simulink model "threephaseinverter_SRF"  (R2023b)
settings: Solver=VariableStepAuto  StartTime=0.0  StopTime=30  RelTol=1e-3
libraries: spsGroundLib x13, spsSeriesRLCBranchLib x12, spsBreakerLib x9, spsIGBTDiodeLib x6, spsSeriesRLCLoadLib x6, spsCurrentMeasurementLib x5, spsVoltageMeasurementLib x4, eeGeneralControl x4, dspsigops x3, slpidlib x2, spsAlphaBetaZerotodq0Lib x2, spsabctoAlphaBetaZeroLib x2
settings Model: Creator=Jia Yee Wong  LastModifiedBy=Jia Yee Wong
settings SFSimCC: SimCustomHeaderCode="#include \"referencegen.h\""  SimUserSources=referencegen.cpp;  SimUserIncludeDirs=C:\JJ\FinalYearProject  DefaultCustomCodeDeterministicFunctions=ByFunction  SimTargetLang=C++

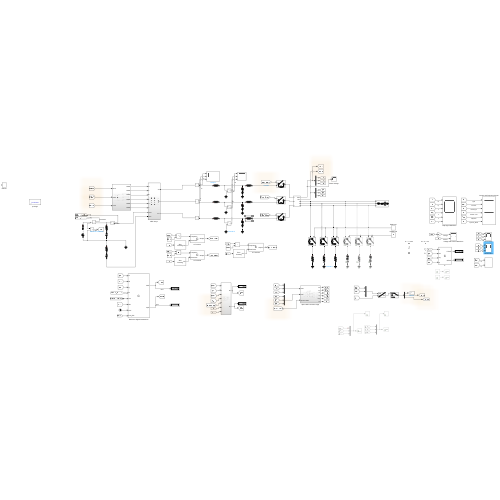
[thumbnail: Simulink's stored preview of the top-level diagram]
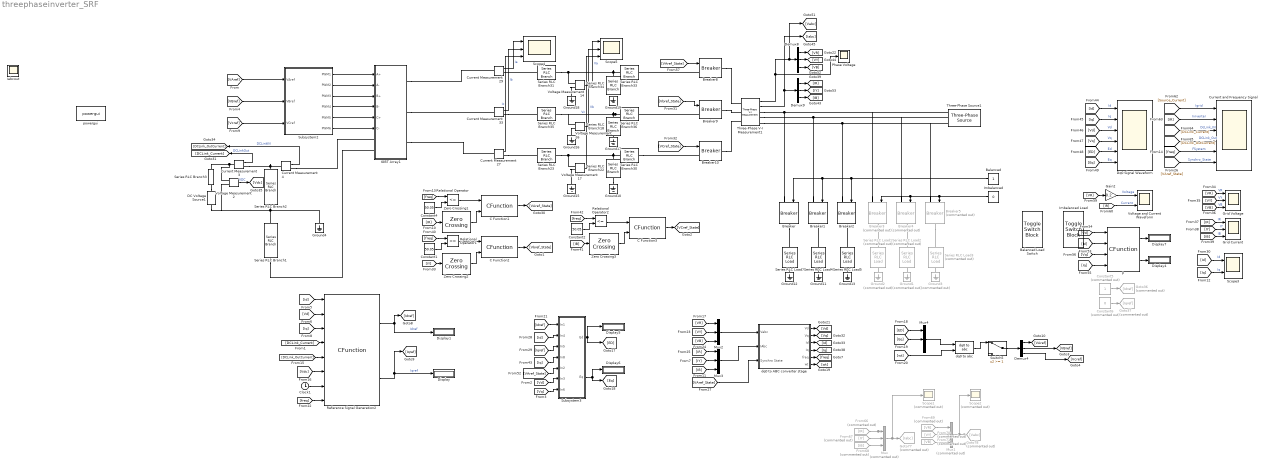
== system threephaseinverter_SRF ==
  Balanced : Constant
  Balanced Load Switch : ToggleSwitchBlock
      settings: Values={{'Off', 'On'}, [0 1]}
  Breaker : spsBreakerLib/Breaker  InitialState=0  SwitchingTimes="[1/60  5/60]"  External=on  BreakerResistance=0.01  SnubberResistance=1e6  SnubberCapacitance=inf  Measurements=None  MoreParameters=on  NoBreakLoop=off
  Breaker1 : spsBreakerLib/Breaker  InitialState=0  SwitchingTimes="[1/60  5/60]"  External=on  BreakerResistance=0.01  SnubberResistance=1e6  SnubberCapacitance=inf  Measurements=None  MoreParameters=on  NoBreakLoop=off
  Breaker10 : spsBreakerLib/Breaker  InitialState=0  SwitchingTimes="[1/60  5/60]"  External=on  BreakerResistance=0.00001  SnubberResistance=30  SnubberCapacitance=47e-9  Measurements=None  MoreParameters=on  NoBreakLoop=off
  Breaker2 : spsBreakerLib/Breaker  InitialState=0  SwitchingTimes="[1/60  5/60]"  External=on  BreakerResistance=0.01  SnubberResistance=1e6  SnubberCapacitance=inf  Measurements=None  MoreParameters=on  NoBreakLoop=off
  Breaker3 : spsBreakerLib/Breaker  Commented=on  InitialState=0  SwitchingTimes="[1/60  5/60]"  External=on  BreakerResistance=0.01  SnubberResistance=1e6  SnubberCapacitance=inf  Measurements=None  MoreParameters=on  NoBreakLoop=off
  Breaker4 : spsBreakerLib/Breaker  Commented=on  InitialState=0  SwitchingTimes="[1/60  5/60]"  External=on  BreakerResistance=0.01  SnubberResistance=1e6  SnubberCapacitance=inf  Measurements=None  MoreParameters=on  NoBreakLoop=off
  Breaker5 : spsBreakerLib/Breaker  Commented=on  InitialState=0  SwitchingTimes="[1/60  5/60]"  External=on  BreakerResistance=0.01  SnubberResistance=1e6  SnubberCapacitance=inf  Measurements=None  MoreParameters=on  NoBreakLoop=off
  Breaker8 : spsBreakerLib/Breaker  InitialState=0  SwitchingTimes="[1/60  5/60]"  External=on  BreakerResistance=0.00001  SnubberResistance=30  SnubberCapacitance=47e-9  Measurements=None  MoreParameters=on  NoBreakLoop=off
  Breaker9 : spsBreakerLib/Breaker  InitialState=0  SwitchingTimes="[1/60  5/60]"  External=on  BreakerResistance=0.00001  SnubberResistance=30  SnubberCapacitance=47e-9  Measurements=None  MoreParameters=on  NoBreakLoop=off
  C Function1 : CFunction  OutputCode=|  SampleTime=1/50000
      | if(Frequency == true && ZeroCross == 1){
      |     Output = 1;}
      | else if(Frequency == false){
      |         Output = 0;}
  C Function2 : CFunction  OutputCode=|  SampleTime=1/50000
      | if(Frequency == true && ZeroCross == 1){
      |     Output = 1;}
      | else if(Frequency == false){
      |         Output = 0;}
  C Function3 : CFunction  OutputCode=|  SampleTime=1/50000
      | if(Frequency == true && ZeroCross == 1){
      |     Output = 1;}
      | else if(Frequency == false){
      |         Output = 0;}
  Clock1 : Clock
  Constant1 : Constant  Value=50.05  SampleTime=1/50000
  Constant2 : Constant  Value=50.05  SampleTime=1/50000
  Constant4 : Constant  Value=50.05  SampleTime=1/50000
  Constant5 : Constant  Commented=on
  Constant6 : Constant  Commented=on  Value=0
  Current Measurement{3..4,27,29,33} (5 alike) : spsCurrentMeasurementLib/Current Measurement  PhasorSimulation=off  OutputType=Complex  PSBequivalent=0
  Current and Frequency Signal : Scope  NumInputPorts=6
  DC Voltage Source1 : spsDCVoltageSourceLib/DC Voltage Source  Amplitude=400  Measurements=None
  Demux4 : Demux  Outputs=3
  Demux8 : Demux  Outputs=3
  Demux9 : Demux  Outputs=3
  Display{,1,4..7} (6 alike) : Display
  Dq0 Signal Waveform : Scope  NumInputPorts=6
  From66 : From  Commented=on  GotoTag=IR
  From67 : From  Commented=on  GotoTag=IY
  From68 : From  Commented=on  GotoTag=IB
  From69 : From  Commented=on  GotoTag=VR
  From70 : From  Commented=on  GotoTag=VY
  From71 : From  Commented=on  GotoTag=VB
  Gain2 : Gain  Gain=0.2
  Goto36 : Goto  Commented=on  GotoTag=Idref
  Goto37 : Goto  Commented=on  GotoTag=Iqref
  Goto77 : Goto  Commented=on  GotoTag=Iabc
  Goto78 : Goto  Commented=on  GotoTag=Vabc
  Grid Current : Scope  NumInputPorts=3
  Grid Voltage : Scope  NumInputPorts=3
  Ground1 : spsGroundLib/Ground  Commented=on  LConnTagsString=a
  Ground{4,10..13,15..19} (10 alike) : spsGroundLib/Ground  LConnTagsString=a
  Ground2 : spsGroundLib/Ground  Commented=on  LConnTagsString=a
  Ground3 : spsGroundLib/Ground  Commented=on  LConnTagsString=a
  IGBT Array1 : Subsystem
  Iabcout : Scope
  Imbalanced : Constant  Value=0
  Imbalanced Load : ToggleSwitchBlock
      settings: Values={{'Off', 'On'}, [0 1]}
  Mux : Mux  Commented=on  Inputs=3
  Mux1 : Mux  Commented=on  Inputs=3
  Mux2 : Mux  Inputs=3
  Mux3 : Mux  Inputs=3
  Mux4 : Mux  Inputs=3
  P : CFunction  OutputCode=|
      | PTotal = Id*Vd;
      | QTotal = Id*Vq-Vq*Id;
  Phase Voltage : Scope
  Reference Signal Generation2 : CFunction  OutputCode=|  StartCode=|  SampleTime=1/50000
      OutputCode=|
      | if(Id!=PreviousId || Iq!=PreviousIq){
      |     if(ReferenceGenTrigger(Freq_PLL)){
      |         Idref=IdrefCalc(CLK,Vd,Iin,Iout, Vdc, Vdc);
      |   //Idref =1;
      |    Iqref=0;
      |    PreviousId=Id;
      |    PreviousIq=Iq;
      |    }
      |   
      | } else { Idref = 0; Iqref = 0;}
      StartCode=|
      | PreviousIq =0;
      | PreviousId =0;
  Relational Operator : RelationalOperator  Operator=<=  OutDataTypeStr=boolean  RndMeth=Simplest  InputSameDT=off
  Relational Operator1 : RelationalOperator  Operator=<=  OutDataTypeStr=boolean  RndMeth=Simplest  InputSameDT=off
  Relational Operator2 : RelationalOperator  Operator=<=  OutDataTypeStr=boolean  RndMeth=Simplest  InputSameDT=off
  Scope1 : Scope  Commented=on
  Scope2 : Scope  Commented=on
  Scope3 : Scope  NumInputPorts=2
  Scope4 : Scope  NumInputPorts=3
  Scope5 : Scope  NumInputPorts=3
  Series RLC Branch1 : spsSeriesRLCBranchLib/Series RLC Branch  LConnTagsString=__new0  RConnTagsString=__new0  BranchType=RC  Resistance=1  Inductance=0  SetiL0=off  InitialCurrent=0  Capacitance=47e-3  Setx0=off  InitialVoltage=300  Measurements=None
  Series RLC Branch18 : spsSeriesRLCBranchLib/Series RLC Branch  LConnTagsString=__new0  RConnTagsString=__new0  BranchType=RC  Resistance=120  Inductance=100e-6  SetiL0=off  InitialCurrent=0  Capacitance=5.526e-6  Setx0=off  InitialVoltage=0  Measurements=None
  Series RLC Branch2 : spsSeriesRLCBranchLib/Series RLC Branch  LConnTagsString=__new0  RConnTagsString=__new0  BranchType=RC  Resistance=1  Inductance=0  SetiL0=off  InitialCurrent=0  Capacitance=47e-3  Setx0=off  InitialVoltage=300  Measurements=None
  Series RLC Branch22 : spsSeriesRLCBranchLib/Series RLC Branch  LConnTagsString=__new0  RConnTagsString=__new0  BranchType=RC  Resistance=120  Inductance=100e-6  SetiL0=off  InitialCurrent=0  Capacitance=5.526e-6  Setx0=off  InitialVoltage=0  Measurements=None
  Series RLC Branch23 : spsSeriesRLCBranchLib/Series RLC Branch  LConnTagsString=__new0  RConnTagsString=__new0  BranchType=L  Resistance=1  Inductance=20.4e-3  SetiL0=off  InitialCurrent=0  Capacitance=1e-6  Setx0=off  InitialVoltage=0  Measurements=None
  Series RLC Branch3 : spsSeriesRLCBranchLib/Series RLC Branch  LConnTagsString=__new0  RConnTagsString=__new0  BranchType=RL  Resistance=100  Inductance=0  SetiL0=off  InitialCurrent=0  Capacitance=1e-6  Setx0=off  InitialVoltage=0  Measurements=None
  Series RLC Branch30 : spsSeriesRLCBranchLib/Series RLC Branch  LConnTagsString=__new0  RConnTagsString=__new0  BranchType=L  Resistance=1  Inductance=148.336e-6  SetiL0=off  InitialCurrent=0  Capacitance=1e-6  Setx0=off  InitialVoltage=0  Measurements=None
  Series RLC Branch31 : spsSeriesRLCBranchLib/Series RLC Branch  LConnTagsString=__new0  RConnTagsString=__new0  BranchType=L  Resistance=1  Inductance=20.4e-3  SetiL0=off  InitialCurrent=0  Capacitance=1e-6  Setx0=off  InitialVoltage=0  Measurements=None
  Series RLC Branch33 : spsSeriesRLCBranchLib/Series RLC Branch  LConnTagsString=__new0  RConnTagsString=__new0  BranchType=L  Resistance=1  Inductance=148.336e-6  SetiL0=off  InitialCurrent=0  Capacitance=1e-6  Setx0=off  InitialVoltage=0  Measurements=None
  Series RLC Branch34 : spsSeriesRLCBranchLib/Series RLC Branch  LConnTagsString=__new0  RConnTagsString=__new0  BranchType=RC  Resistance=120  Inductance=100e-6  SetiL0=off  InitialCurrent=0  Capacitance=5.526e-6  Setx0=off  InitialVoltage=0  Measurements=None
  Series RLC Branch35 : spsSeriesRLCBranchLib/Series RLC Branch  LConnTagsString=__new0  RConnTagsString=__new0  BranchType=L  Resistance=1  Inductance=20.4e-3  SetiL0=off  InitialCurrent=0  Capacitance=1e-6  Setx0=off  InitialVoltage=0  Measurements=None
  Series RLC Branch36 : spsSeriesRLCBranchLib/Series RLC Branch  LConnTagsString=__new0  RConnTagsString=__new0  BranchType=L  Resistance=1  Inductance=148.336e-6  SetiL0=off  InitialCurrent=0  Capacitance=1e-6  Setx0=off  InitialVoltage=0  Measurements=None
  Series RLC Load1 : spsSeriesRLCLoadLib/Series RLC Load  Commented=on  LConnTagsString=a  RConnTagsString=__new0  NominalVoltage=240  NominalFrequency=50  ActivePower=10e3  InductivePower=300  CapacitivePower=200  Setx0=off  InitialVoltage=240  SetiL0=off  InitialCurrent=10  Measurements=None  LoadType=constant PQ
  Series RLC Load2 : spsSeriesRLCLoadLib/Series RLC Load  Commented=on  LConnTagsString=a  RConnTagsString=__new0  NominalVoltage=240  NominalFrequency=50  ActivePower=10e3  InductivePower=0  CapacitivePower=0  Setx0=off  InitialVoltage=240  SetiL0=off  InitialCurrent=10  Measurements=None  LoadType=constant PQ
  Series RLC Load3 : spsSeriesRLCLoadLib/Series RLC Load  Commented=on  LConnTagsString=a  RConnTagsString=__new0  NominalVoltage=240  NominalFrequency=50  ActivePower=5e3  InductivePower=400  CapacitivePower=0  Setx0=off  InitialVoltage=240  SetiL0=off  InitialCurrent=10  Measurements=None  LoadType=constant PQ
  Series RLC Load4 : spsSeriesRLCLoadLib/Series RLC Load  LConnTagsString=a  RConnTagsString=__new0  NominalVoltage=240  NominalFrequency=50  ActivePower=10e2  InductivePower=0  CapacitivePower=0  Setx0=off  InitialVoltage=240  SetiL0=off  InitialCurrent=10  Measurements=None  LoadType=constant PQ
  Series RLC Load5 : spsSeriesRLCLoadLib/Series RLC Load  LConnTagsString=a  RConnTagsString=__new0  NominalVoltage=240  NominalFrequency=50  ActivePower=10e2  InductivePower=0  CapacitivePower=0  Setx0=off  InitialVoltage=240  SetiL0=off  InitialCurrent=10  Measurements=None  LoadType=constant PQ
  Series RLC Load7 : spsSeriesRLCLoadLib/Series RLC Load  LConnTagsString=a  RConnTagsString=__new0  NominalVoltage=240  NominalFrequency=50  ActivePower=10e2  InductivePower=0  CapacitivePower=0  Setx0=off  InitialVoltage=240  SetiL0=off  InitialCurrent=10  Measurements=None  LoadType=constant PQ
  Subsystem2 : Subsystem
  Subsystem3 : Subsystem
  Switch5 : Switch  Threshold=1  SaturateOnIntegerOverflow=off  InputSameDT=off
  Three-Phase V-I Measurement1 : spsThreePhaseVIMeasurementLib/Three-Phase V-I Measurement  VoltageMeasurement=phase-to-phase  SetLabelV=off  LabelV=Vabc  Vpu=off  VpuLL=off  CurrentMeasurement=yes  SetLabelI=off  LabelI=Iabc  Ipu=off  Pbase=100e6  Vbase=500e3  OutputType=Complex  PhasorSimulation=off  PSBequivalent=0
  Three-Phase Source1 : spsThreePhaseSourceLib/Three-Phase Source  InternalConnection=Yg  VoltagePhases=off  Voltage=240  PhaseAngle=0  Voltage_phases=[25e3 25e3 25e3]/sqrt(3)  PhaseAngles_phases=[0 -120 +120]  Frequency=50  NonIdealSource=on  SpecifyImpedance=off  Resistance=0.001E-3  Inductance=0.001E-3  ShortCircuitLevel=100e6  BaseVoltage=240  XRratio=7  BusType=PQ  Pref=1000  Qref=0  Prefabc=[10e3, 10e3, 10e3]  Qrefabc=[0, 0, 0]  Qmin=-inf  Qmax=inf
  Voltage Measurement{2,14,16..17} (4 alike) : spsVoltageMeasurementLib/Voltage Measurement  PhasorSimulation=off  OutputType=Complex  PSBequivalent=0
  Voltage and Current Waveform : Scope  NumInputPorts=2
  Zero Crossing1 : dspsigops/Zero Crossing
  Zero Crossing2 : dspsigops/Zero Crossing
  Zero Crossing3 : dspsigops/Zero Crossing
  dq0 to ABC converter stage : Subsystem
  dq0 to abc : spsdq0toabcLib/dq0 to abc  Alignment=90 degrees behind phase A axis
  powergui : spspowerguiLib/powergui  Priority=1  SimulationMode=Continuous  SampleTime=50e-6  frequency=60  Iterations=50  frequencyindice=0  Pbase=100e6  ErrMax=1e-4  UnitsV=kV  UnitsW=MW  buscounter=0  FunctionMessages=off  echomessages=off  EnableUseOfTLC=off  CurrentSourceSwitches=off  DisableSnubberDevices=off  DisableRonSwitches=off  DisableVfSwitches=off  DisplayEquations=off  AutomaticDiscreteSolvers=off  SolverType=Tustin/Backward Euler (TBE)  Interpol=off  ExternalGateDelay=off  methode=off  Ts=100  x0status=blocks  SPID=on  SwTol=0  HookPort=off  NonlinearTolerance=1e-4  nMaxIteration=100  ContinueOnMaxIteration=off  RestoreLinks=warning  ResistiveCurrentMeasurement=off  Frange=[0:2:500]  Ylog=off  Xlog=on  ShowGrid=off  save=off  variable=ZData  structure=0  ZoomFFT=off  StartTime=0.0  cycles=1  DisplayStyle=1  fundamental=60  FreqAxis=off  MaxFrequency=1000  frequencyindicesteady=1  RmsSteady=1  display=off
  wires:
  Mux/1 -> Scope1/1, Goto77/1
  From68/1 -> Mux/3
  From67/1 -> Mux/2
  From66/1 -> Mux/1
  From70/1 -> Mux1/2
  From69/1 -> Mux1/1
  From71/1 -> Mux1/3
  Mux1/1 -> Scope2/1, Goto78/1
  Demux9/3 -> [IB]
  Demux9/1 -> [IR]
  Demux8/2 -> [VY]
  Demux8/1 -> [VR]
  Three-Phase V-I Measurement1/2 -> [Iabc], Demux9/1
  [VAref_State] -> Breaker8/1
  [Vbref_State] -> Breaker9/1
  Three-Phase V-I Measurement1/1 -> Phase Voltage/1, [Vabc], Demux8/1
  Demux8/3 -> [VB]
  Voltage Measurement16/1 -> Scope5/2  "Vb"
  Voltage Measurement14/1 -> Scope5/1  "Va"
  [VCref_State] -> Breaker10/1
  Demux9/2 -> [IY]
  Balanced/1 -> Breaker2/1, Breaker1/1, Breaker/1
  Voltage Measurement17/1 -> Scope5/3  "Vc"
  Imbalanced/1 -> Breaker5/1, Breaker4/1, Breaker3/1
  Current Measurement27/1 -> Scope4/3  "Ic"
  Current Measurement33/1 -> Scope4/2  "Ib"
  Current Measurement29/1 -> Scope4/1  "Ia"
  Subsystem2/1(PWM1) -> IGBT Array1/1(A+)
  Subsystem2/2(PWM2) -> IGBT Array1/2(A-)
  Subsystem2/3(PWM3) -> IGBT Array1/3(B+)
  Subsystem2/4(PWM4) -> IGBT Array1/4(B-)
  Subsystem2/5(PWM5) -> IGBT Array1/5(C+)
  Subsystem2/6(PWM6) -> IGBT Array1/6(C-)
  Current Measurement4/1 -> [DCLink_OutCurrent]  "DCLinkIN"
  Current Measurement3/1 -> [DCLink_Current]  "DCLinkOut"
  Voltage Measurement2/1 -> [Vdc]  "VDC"
  Reference Signal Generation2/1 -> Display1/1, [Idref]  "Idref"
  [Id] -> Reference Signal Generation2/1
  Clock1/1 -> Reference Signal Generation2/7
  [freq] -> Reference Signal Generation2/8
  [Iq] -> Reference Signal Generation2/3
  [DCLink_OutCurrent] -> Reference Signal Generation2/5
  [Vdc] -> Reference Signal Generation2/6
  [Vd] -> Reference Signal Generation2/2
  [DCLink_Current] -> Reference Signal Generation2/4
  Reference Signal Generation2/2 -> [Iqref], Display/1  "Iqref"
  [Id] -> Subsystem3/2(In4)
  [VAref_State] -> Subsystem3/5(In2)
  [Iq] -> Subsystem3/4(In8)
  Subsystem3/2(Eq) -> [Eq], Display6/1
  Subsystem3/1(Ed) -> [ED], Display5/1
  [Vq] -> Subsystem3/7(In6)
  [Vd] -> Subsystem3/6(In3)
  [Iqref] -> Subsystem3/3(In5)
  [Idref] -> Subsystem3/1(In1)
  Mux3/1 -> dq0 to ABC converter stage/2(IAbc)
  [VB] -> Mux2/3
  dq0 to ABC converter stage/4(Iq) -> [Iq]
  [IB] -> Mux3/3
  dq0 to ABC converter stage/3(Id) -> [Id]
  dq0 to ABC converter stage/5(freq) -> [freq]
  [IR] -> Mux3/1
  dq0 to ABC converter stage/2(Vq) -> [Vq]
  Mux2/1 -> dq0 to ABC converter stage/1(Vabc)
  dq0 to ABC converter stage/1(Vd) -> [Vd]
  [VR] -> Mux2/1
  [IY] -> Mux3/2
  [VAref_State] -> dq0 to ABC converter stage/3(Synchro State)
  dq0 to ABC converter stage/6(wt) -> [wt]
  [VY] -> Mux2/2
  Switch5/1 -> Demux4/1
  [ED] -> Mux4/1
  Mux4/1 -> dq0 to abc/1
  dq0 to abc/1 -> Switch5/1
  [Eq] -> Mux4/2
  [wt] -> dq0 to abc/2
  Demux4/1 -> [VAref]
  Demux4/2 -> [VBref]
  Demux4/3 -> [Vcref]
  [Vcref] -> Subsystem2/3(VCref)
  [VBref] -> Subsystem2/2(VBref)
  [VAref] -> Subsystem2/1(VAref)
  Zero Crossing1/1 -> C Function1/2
  Constant4/1 -> Relational Operator/2
  [IR] -> Zero Crossing1/1
  Relational Operator/1 -> C Function1/1
  [freq] -> Relational Operator/1
  C Function1/1 -> [VAref_State]
  P/2 -> Display4/1
  [freq] -> Current and Frequency Signal/5  "FSystem"
  Constant5/1 -> Goto36/1
  [IR] -> Grid Current/1  "IR"
  P/1 -> Display7/1
  Constant6/1 -> Goto37/1
  [IB] -> Grid Current/3  "IB"
  [ED] -> Dq0 Signal Waveform/5  "Ed"
  [VAref_State] -> Current and Frequency Signal/6  "Synchro_State"
  [Id] -> P/2
  [DCLink_Current] -> Current and Frequency Signal/3  "DcLink_IN"
  [Vq] -> Dq0 Signal Waveform/4  "Vq"
  [VR] -> Grid Voltage/1  "VR"
  [Vd] -> Dq0 Signal Waveform/3  "Vd"
  [VR] -> Gain2/1
  [VY] -> Grid Voltage/2  "VY"
  [Vd] -> P/1
  [IR] -> Voltage and Current Waveform/2  "Current"
  [IY] -> Grid Current/2  "IY"
  [Vq] -> P/3
  [Eq] -> Dq0 Signal Waveform/6  "Eq"
  [IR] -> Current and Frequency Signal/2  "Iinverter"
  Gain2/1 -> Voltage and Current Waveform/1  "Voltage"
  [Source_Current] -> Current and Frequency Signal/1  "Igrid"
  [Iq] -> Dq0 Signal Waveform/2  "Iq"
  [VB] -> Grid Voltage/3  "VB"
  [Iq] -> Scope3/2  "Iq"
  [Id] -> Scope3/1  "Id"
  [Id] -> Dq0 Signal Waveform/1  "Id"
  [DCLink_OutCurrent] -> Current and Frequency Signal/4  "DCLink_Out"
  [Iq] -> P/4
  C Function2/1 -> [Vbref_State]
  Zero Crossing2/1 -> C Function2/2
  Constant1/1 -> Relational Operator1/2
  Relational Operator1/1 -> C Function2/1
  [IY] -> Zero Crossing2/1
  [freq] -> Relational Operator1/1
  [freq] -> Relational Operator2/1
  Zero Crossing3/1 -> C Function3/2
  Relational Operator2/1 -> C Function3/1
  [IB] -> Zero Crossing3/1
  Constant2/1 -> Relational Operator2/2
  C Function3/1 -> [VCref_State]
  connections:
  Three-Phase V-I Measurement1/RConn3 -- Three-Phase Source1/RConn3 -- Breaker5/LConn1 -- Breaker2/LConn1
  Three-Phase V-I Measurement1/RConn1 -- Three-Phase Source1/RConn1 -- Breaker3/LConn1 -- Breaker/LConn1
  Voltage Measurement17/LConn1 -- Series RLC Branch23/RConn1 -- Series RLC Branch30/LConn1 -- Series RLC Branch22/LConn1
  Voltage Measurement14/LConn1 -- Series RLC Branch31/RConn1 -- Series RLC Branch33/LConn1 -- Series RLC Branch34/LConn1
  Three-Phase V-I Measurement1/RConn2 -- Three-Phase Source1/RConn2 -- Breaker4/LConn1 -- Breaker1/LConn1
  Series RLC Branch36/LConn1 -- Voltage Measurement16/LConn1 -- Series RLC Branch35/RConn1 -- Series RLC Branch18/LConn1
  Breaker9/LConn1 -- Series RLC Branch36/RConn1
  Voltage Measurement17/LConn2 -- Ground15/LConn1
  Breaker8/LConn1 -- Series RLC Branch33/RConn1
  Ground12/LConn1 -- Series RLC Load7/RConn1
  Ground16/LConn1 -- Voltage Measurement16/LConn2
  Breaker8/RConn1 -- Three-Phase V-I Measurement1/LConn1
  Voltage Measurement14/LConn2 -- Ground18/LConn1
  Breaker9/RConn1 -- Three-Phase V-I Measurement1/LConn2
  Series RLC Load4/RConn1 -- Ground11/LConn1
  Series RLC Branch30/RConn1 -- Breaker10/LConn1
  Series RLC Branch22/RConn1 -- Ground10/LConn1
  Series RLC Load5/RConn1 -- Ground13/LConn1
  Breaker10/RConn1 -- Three-Phase V-I Measurement1/LConn3
  Current Measurement29/RConn1 -- Series RLC Branch31/LConn1
  Series RLC Branch18/RConn1 -- Ground17/LConn1
  IGBT Array1/RConn2 -- Current Measurement33/LConn1
  Current Measurement27/RConn1 -- Series RLC Branch23/LConn1
  Current Measurement33/RConn1 -- Series RLC Branch35/LConn1
  IGBT Array1/RConn3 -- Current Measurement27/LConn1
  Breaker/RConn1 -- Series RLC Load7/LConn1
  Series RLC Load4/LConn1 -- Breaker1/RConn1
  Series RLC Load5/LConn1 -- Breaker2/RConn1
  Ground2/LConn1 -- Series RLC Load1/RConn1
  Ground1/LConn1 -- Series RLC Load2/RConn1
  Breaker3/RConn1 -- Series RLC Load1/LConn1
  Ground3/LConn1 -- Series RLC Load3/RConn1
  Breaker4/RConn1 -- Series RLC Load2/LConn1
  Breaker5/RConn1 -- Series RLC Load3/LConn1
  IGBT Array1/RConn1 -- Current Measurement29/LConn1
  Series RLC Branch2/LConn1 -- Current Measurement4/LConn1 -- Current Measurement3/RConn1
  Series RLC Branch2/RConn1 -- Ground4/LConn1 -- Series RLC Branch1/LConn1 -- Voltage Measurement2/LConn2 -- DC Voltage Source1/LConn1
  Voltage Measurement2/LConn1 -- Series RLC Branch3/LConn1 -- Current Measurement3/LConn1
  Current Measurement4/RConn1 -- IGBT Array1/LConn1
  Series RLC Branch3/RConn1 -- DC Voltage Source1/RConn1
  Series RLC Branch1/RConn1 -- IGBT Array1/LConn2

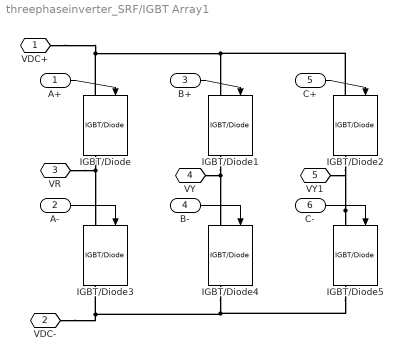
== system threephaseinverter_SRF/IGBT Array1 ==
  A+ : Inport
  A- : Inport  Port=2
  B+ : Inport  Port=3
  B- : Inport  Port=4
  C+ : Inport  Port=5
  C- : Inport  Port=6
  IGBT/Diode{,1..5} (6 alike) : spsIGBTDiodeLib/IGBT//Diode  Ron=1e-3  Rs=1e5  Cs=inf  Measurements=on
  VDC+ : PMIOPort  Side=Left
  VDC- : PMIOPort  Port=2  Side=Left
  VR : PMIOPort  Port=3  Side=Right
  VY : PMIOPort  Port=4  Side=Right
  VY1 : PMIOPort  Port=5  Side=Right
  wires:
  A-/1 -> IGBT/Diode3/1
  B-/1 -> IGBT/Diode4/1
  B+/1 -> IGBT/Diode1/1
  A+/1 -> IGBT/Diode/1
  C+/1 -> IGBT/Diode2/1
  C-/1 -> IGBT/Diode5/1
  connections:
  IGBT/Diode4/RConn1 -- IGBT/Diode5/RConn1 -- VDC-/RConn1 -- IGBT/Diode3/RConn1
  IGBT/Diode/RConn1 -- VR/RConn1 -- IGBT/Diode3/LConn1
  IGBT/Diode1/RConn1 -- VY/RConn1 -- IGBT/Diode4/LConn1
  IGBT/Diode/LConn1 -- VDC+/RConn1 -- IGBT/Diode2/LConn1 -- IGBT/Diode1/LConn1
  IGBT/Diode5/LConn1 -- IGBT/Diode2/RConn1 -- VY1/RConn1

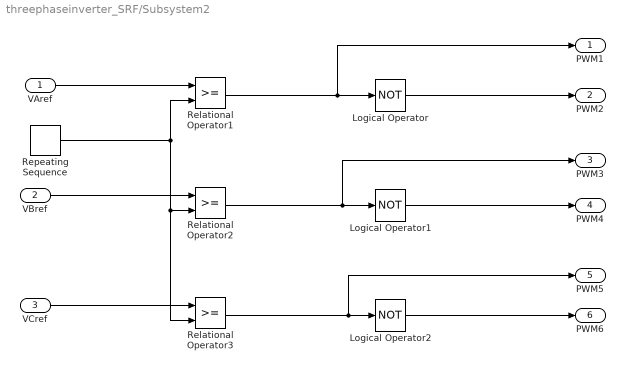
== system threephaseinverter_SRF/Subsystem2 ==
  VAref : Inport
  VBref : Inport  Port=2
  VCref : Inport  Port=3
  Logical Operator : Logic  Operator=NOT  AllPortsSameDT=off  OutDataTypeStr=boolean
  Logical Operator1 : Logic  Operator=NOT  AllPortsSameDT=off  OutDataTypeStr=boolean
  Logical Operator2 : Logic  Operator=NOT  AllPortsSameDT=off  OutDataTypeStr=boolean
  Relational Operator1 : RelationalOperator  OutDataTypeStr=boolean  RndMeth=Simplest  InputSameDT=off
  Relational Operator2 : RelationalOperator  OutDataTypeStr=boolean  RndMeth=Simplest  InputSameDT=off
  Relational Operator3 : RelationalOperator  OutDataTypeStr=boolean  RndMeth=Simplest  InputSameDT=off
  Repeating Sequence : simulink/Sources/Repeating Sequence  rep_seq_t=[0 0.00005 0.0001]  rep_seq_y=[-1 1 -1]
  PWM1 : Outport
  PWM2 : Outport  Port=2
  PWM3 : Outport  Port=3
  PWM4 : Outport  Port=4
  PWM5 : Outport  Port=5
  PWM6 : Outport  Port=6
  wires:
  Logical Operator2/1 -> PWM6/1
  Repeating Sequence/1 -> Relational Operator1/2, Relational Operator3/2, Relational Operator2/2
  VBref/1 -> Relational Operator2/1
  Logical Operator1/1 -> PWM4/1
  VCref/1 -> Relational Operator3/1
  VAref/1 -> Relational Operator1/1
  Logical Operator/1 -> PWM2/1
  Relational Operator1/1 -> PWM1/1, Logical Operator/1
  Relational Operator2/1 -> PWM3/1, Logical Operator1/1
  Relational Operator3/1 -> PWM5/1, Logical Operator2/1

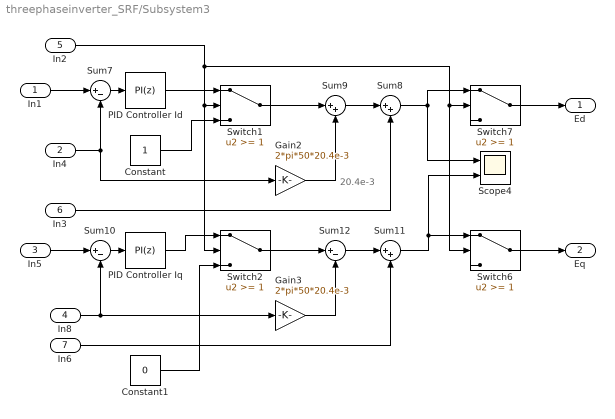
== system threephaseinverter_SRF/Subsystem3 ==
  note: 20.4e-3
  In1 : Inport
  In4 : Inport  Port=2
  In5 : Inport  Port=3
  In8 : Inport  Port=4
  In2 : Inport  Port=5
  In3 : Inport  Port=6
  In6 : Inport  Port=7
  Constant : Constant
  Constant1 : Constant  Value=0
  Gain2 : Gain  Gain=2*pi*50*20.4e-3
  Gain3 : Gain  Gain=2*pi*50*20.4e-3
  PID Controller Id : slpidlib/PID Controller  Controller=PI  Form=Parallel  TimeDomain=Discrete-time  UseExternalTs=off  SampleTime=5e-5  IntegratorMethod=Forward Euler  FilterMethod=Forward Euler  ControllerParametersSource=internal  P=0.25  I=0.2  UseKiTs=on  D=0.2  N=100  UseFilter=on  TunerSelectOption=Transfer Function Based (PID Tuner App)  InitialConditionSource=internal  InitialConditionForIntegrator=0  InitialConditionForFilter=0  DifferentiatorICPrevScaledInput=0  ExternalReset=none  TrackingMode=off  Kt=1  LimitOutput=on  SatLimitsSource=internal  UpperSaturationLimit=200  LowerSaturationLimit=-200  LinearizeAsGain=on  AntiWindupMode=back-calculation  Kb=1  LimitIntegrator=off  UpperIntegratorSaturationLimit=inf  LowerIntegratorSaturationLimit=-inf  POutMin=[]  POutMax=[]  IOutMin=[]  IOutMax=[]  DOutMin=[]  DOutMax=[]  NOutMin=[]  NOutMax=[]  SumOutMin=[]  SumOutMax=[]  SaturationOutMin=[]  SaturationOutMax=[]  PParamMin=[]  PParamMax=[]  IParamMin=[]  IParamMax=[]  DParamMin=[]  DParamMax=[]  NParamMin=[]  NParamMax=[]  KbParamMin=[]  KbParamMax=[]  KtParamMin=[]  KtParamMax=[]  KbOutMin=[]  KbOutMax=[]  KtOutMin=[]  KtOutMax=[]  IntegratorOutMin=[]  IntegratorOutMax=[]  FilterOutMin=[]  FilterOutMax=[]  SumI1OutMin=[]  SumI1OutMax=[]  SumI2OutMin=[]  SumI2OutMax=[]  SumI3OutMin=[]  SumI3OutMax=[]  SumI4OutMin=[]  SumI4OutMax=[]  SumDOutMin=[]  SumDOutMax=[]  DifferentiatorOutMin=[]  DifferentiatorOutMax=[]  FilterDiffOutCoefMin=[]  FilterDiffOutCoefMax=[]  ReciprocalOutMin=[]  ReciprocalOutMax=[]  SumDenOutMin=[]  SumDenOutMax=[]  SumNumOutMin=[]  SumNumOutMax=[]  DivideOutMin=[]  DivideOutMax=[]  UdiffTsProdOutMin=[]  UdiffTsProdOutMax=[]  NTsProdOutMin=[]  NTsProdOutMax=[]  UintegralTsProdOutMin=[]  UintegralTsProdOutMax=[]  UngainTsProdOutMin=[]  UngainTsProdOutMax=[]  ClampingZeroOutDataTypeStr=Inherit: Inherit via back propagation  ClampingZeroOutMin=[]  ClampingZeroOutMax=[]  FilterDenConstantOutDataTypeStr=Inherit: Inherit via back propagation  FilterDenConstantOutMin=[]  FilterDenConstantOutMax=[]  PCopyOutDataTypeStr=Inherit: Inherit via back propagation  PCopyOutMin=[]  PCopyOutMax=[]  NCopyOutDataTypeStr=Inherit: Inherit via back propagation  NCopyOutMin=[]  NCopyOutMax=[]  IntegratorContinuousStateAttributes=''  IntegratorStateIdentifier=Id  IntegratorStateMustResolveToSignalObject=off  IntegratorRTWStateStorageClass=Auto  FilterContinuousStateAttributes=''  FilterStateMustResolveToSignalObject=off  FilterRTWStateStorageClass=Auto  ParallelPVariant=InternalParameters  IdealPVariant=Disabled  IVariant=InternalParameters  DVariant=Disabled  IntegratorVariant=Discrete  SatVariant=Enabled  AWVariant=BackCalculation  PCopyVariant=Disabled  TRVariant=Disabled  FdbkBlocksVariant=Forward  IdealPFdbkVariant=Disabled  SatFdbkVariant=Disabled  DerivativeFilterVariant=Disabled  NVariant=Disabled  NCopyVariant=Disabled_SignalSpec  FilterICVariant=Disabled  IntegratorICVariant=InternalICs  ExternalResetVariant=Disabled  TRSumVariant=Passthrough  SumFdbkVariant=Disabled  SumVariant=Sum_PI  TsampFilterVariant=InternalTs  TsampNgainVariant=Passthrough  TsampIntegralVariant=Disabled_SignalSpec  ExternalSaturationOutDataTypeStr=Inherit: Same as second input
  PID Controller Iq : slpidlib/PID Controller  Controller=PI  Form=Parallel  TimeDomain=Discrete-time  UseExternalTs=off  SampleTime=5e-5  IntegratorMethod=Forward Euler  FilterMethod=Forward Euler  ControllerParametersSource=internal  P=0.25  I=0.2  UseKiTs=on  D=0.2  N=100  UseFilter=on  TunerSelectOption=Transfer Function Based (PID Tuner App)  InitialConditionSource=internal  InitialConditionForIntegrator=0  InitialConditionForFilter=0  DifferentiatorICPrevScaledInput=0  ExternalReset=none  TrackingMode=off  Kt=1  LimitOutput=on  SatLimitsSource=internal  UpperSaturationLimit=200  LowerSaturationLimit=-200  LinearizeAsGain=on  AntiWindupMode=back-calculation  Kb=1  LimitIntegrator=off  UpperIntegratorSaturationLimit=inf  LowerIntegratorSaturationLimit=-inf  POutMin=[]  POutMax=[]  IOutMin=[]  IOutMax=[]  DOutMin=[]  DOutMax=[]  NOutMin=[]  NOutMax=[]  SumOutMin=[]  SumOutMax=[]  SaturationOutMin=[]  SaturationOutMax=[]  PParamMin=[]  PParamMax=[]  IParamMin=[]  IParamMax=[]  DParamMin=[]  DParamMax=[]  NParamMin=[]  NParamMax=[]  KbParamMin=[]  KbParamMax=[]  KtParamMin=[]  KtParamMax=[]  KbOutMin=[]  KbOutMax=[]  KtOutMin=[]  KtOutMax=[]  IntegratorOutMin=[]  IntegratorOutMax=[]  FilterOutMin=[]  FilterOutMax=[]  SumI1OutMin=[]  SumI1OutMax=[]  SumI2OutMin=[]  SumI2OutMax=[]  SumI3OutMin=[]  SumI3OutMax=[]  SumI4OutMin=[]  SumI4OutMax=[]  SumDOutMin=[]  SumDOutMax=[]  DifferentiatorOutMin=[]  DifferentiatorOutMax=[]  FilterDiffOutCoefMin=[]  FilterDiffOutCoefMax=[]  ReciprocalOutMin=[]  ReciprocalOutMax=[]  SumDenOutMin=[]  SumDenOutMax=[]  SumNumOutMin=[]  SumNumOutMax=[]  DivideOutMin=[]  DivideOutMax=[]  UdiffTsProdOutMin=[]  UdiffTsProdOutMax=[]  NTsProdOutMin=[]  NTsProdOutMax=[]  UintegralTsProdOutMin=[]  UintegralTsProdOutMax=[]  UngainTsProdOutMin=[]  UngainTsProdOutMax=[]  ClampingZeroOutDataTypeStr=Inherit: Inherit via back propagation  ClampingZeroOutMin=[]  ClampingZeroOutMax=[]  FilterDenConstantOutDataTypeStr=Inherit: Inherit via back propagation  FilterDenConstantOutMin=[]  FilterDenConstantOutMax=[]  PCopyOutDataTypeStr=Inherit: Inherit via back propagation  PCopyOutMin=[]  PCopyOutMax=[]  NCopyOutDataTypeStr=Inherit: Inherit via back propagation  NCopyOutMin=[]  NCopyOutMax=[]  IntegratorContinuousStateAttributes=''  IntegratorStateIdentifier=Id  IntegratorStateMustResolveToSignalObject=off  IntegratorRTWStateStorageClass=Auto  FilterContinuousStateAttributes=''  FilterStateMustResolveToSignalObject=off  FilterRTWStateStorageClass=Auto  ParallelPVariant=InternalParameters  IdealPVariant=Disabled  IVariant=InternalParameters  DVariant=Disabled  IntegratorVariant=Discrete  SatVariant=Enabled  AWVariant=BackCalculation  PCopyVariant=Disabled  TRVariant=Disabled  FdbkBlocksVariant=Forward  IdealPFdbkVariant=Disabled  SatFdbkVariant=Disabled  DerivativeFilterVariant=Disabled  NVariant=Disabled  NCopyVariant=Disabled_SignalSpec  FilterICVariant=Disabled  IntegratorICVariant=InternalICs  ExternalResetVariant=Disabled  TRSumVariant=Passthrough  SumFdbkVariant=Disabled  SumVariant=Sum_PI  TsampFilterVariant=InternalTs  TsampNgainVariant=Passthrough  TsampIntegralVariant=Disabled_SignalSpec  ExternalSaturationOutDataTypeStr=Inherit: Same as second input
  Scope4 : Scope  NumInputPorts=2
  Sum10 : Sum  Inputs=|+-
  Sum11 : Sum  Inputs=|++
  Sum12 : Sum  Inputs=|+-
  Sum7 : Sum  Inputs=|+-
  Sum8 : Sum  Inputs=|++
  Sum9 : Sum  Inputs=|++
  Switch{1..2,6..7} (4 alike) : Switch  Threshold=1  SaturateOnIntegerOverflow=off  InputSameDT=off
  Ed : Outport
  Eq : Outport  Port=2
  wires:
  Switch1/1 -> Sum9/1
  In5/1 -> Sum10/1
  In1/1 -> Sum7/1
  In6/1 -> Sum11/2
  In2/1 -> Switch6/2, Switch7/2, Switch2/2, Switch1/2
  Switch7/1 -> Ed/1
  Sum8/1 -> Scope4/1, Switch7/1
  Sum10/1 -> PID Controller Iq/1
  Sum11/1 -> Switch6/1, Scope4/2
  Gain3/1 -> Sum12/2
  Sum7/1 -> PID Controller Id/1
  PID Controller Iq/1 -> Switch2/1
  In3/1 -> Sum8/2
  Sum9/1 -> Sum8/1
  Gain2/1 -> Sum9/2
  Sum12/1 -> Sum11/1
  In4/1 -> Gain2/1, Sum7/2
  In8/1 -> Gain3/1, Sum10/2
  PID Controller Id/1 -> Switch1/1
  Switch2/1 -> Sum12/1
  Switch6/1 -> Eq/1
  Constant/1 -> Switch1/3
  Constant1/1 -> Switch2/3

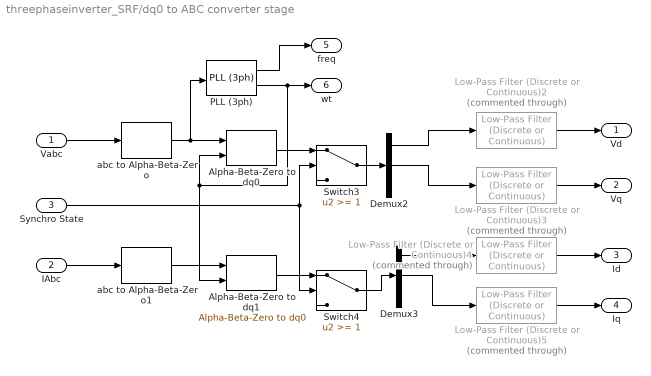
== system threephaseinverter_SRF/dq0 to ABC converter stage ==
  Vabc : Inport
  IAbc : Inport  Port=2
  Synchro State : Inport  Port=3
  Alpha-Beta-Zero to dq0 : spsAlphaBetaZerotodq0Lib/Alpha-Beta-Zero to dq0  Alignment=90 degrees behind phase A axis
  Alpha-Beta-Zero to dq1 : spsAlphaBetaZerotodq0Lib/Alpha-Beta-Zero to dq0  Alignment=90 degrees behind phase A axis
  Demux2 : Demux  Outputs=3
  Demux3 : Demux  Outputs=3
  Low-Pass Filter (Discrete or Continuous){2..5} (4 alike) : eeGeneralControl/Low-Pass Filter (Discrete or Continuous)  Commented=through  K=1  T=2*pi*50  B=inf  A=-inf  init_option=Inherited from block input  x0=0  Ts=0
  PLL (3ph) : spsPLL3phLib/PLL (3ph)  Fmin=45  Par_Init=[0, 60]  ParK=[180, 3200, 1]  TcD=1e-4  MaxRateChangeFreq=12  FilterCutOffFreq=25  Ts=0  AGC=on
  Switch3 : Switch  Threshold=1  SaturateOnIntegerOverflow=off  InputSameDT=off
  Switch4 : Switch  Threshold=1  SaturateOnIntegerOverflow=off  InputSameDT=off
  abc to Alpha-Beta-Zero : spsabctoAlphaBetaZeroLib/abc to Alpha-Beta-Zero
  abc to Alpha-Beta-Zero1 : spsabctoAlphaBetaZeroLib/abc to Alpha-Beta-Zero
  Vd : Outport
  Vq : Outport  Port=2
  Id : Outport  Port=3
  Iq : Outport  Port=4
  freq : Outport  Port=5
  wt : Outport  Port=6
  wires:
  Demux3/2 -> Low-Pass Filter (Discrete or Continuous)5/1
  Synchro State/1 -> Switch4/2, Switch3/2
  Demux3/1 -> Low-Pass Filter (Discrete or Continuous)4/1
  Low-Pass Filter (Discrete or Continuous)5/1 -> Iq/1
  abc to Alpha-Beta-Zero1/1 -> Alpha-Beta-Zero to dq1/1
  Low-Pass Filter (Discrete or Continuous)4/1 -> Id/1
  Switch4/1 -> Demux3/1
  Demux2/2 -> Low-Pass Filter (Discrete or Continuous)3/1
  Low-Pass Filter (Discrete or Continuous)2/1 -> Vd/1
  Alpha-Beta-Zero to dq1/1 -> Switch4/1
  Demux2/1 -> Low-Pass Filter (Discrete or Continuous)2/1
  Low-Pass Filter (Discrete or Continuous)3/1 -> Vq/1
  Switch3/1 -> Demux2/1
  PLL (3ph)/1 -> freq/1
  Alpha-Beta-Zero to dq0/1 -> Switch3/1
  abc to Alpha-Beta-Zero/1 -> PLL (3ph)/1, Alpha-Beta-Zero to dq0/1
  Vabc/1 -> abc to Alpha-Beta-Zero/1
  PLL (3ph)/2 -> Alpha-Beta-Zero to dq1/2, Alpha-Beta-Zero to dq0/2, wt/1
  IAbc/1 -> abc to Alpha-Beta-Zero1/1
